simulink model "Scope1"  (R2025b)
settings: Solver=VariableStepAuto  StartTime=0.0  StopTime=10.0  RelTol=1e-3
libraries: simulink x1
settings Model: Creator=fmarini  LastModifiedBy=Claudia Yasar
settings SolverCC: AlgebraicLoopSolver=TrustRegion
settings DebuggingCC: UnconnectedInputMsg=warning  UnconnectedOutputMsg=warning  UnconnectedLineMsg=warning
settings ModelReferenceCC: EnableRefExpFcnMdlSchedulingChecks=on
settings RTWCC: GPUComputeCapability=3.5

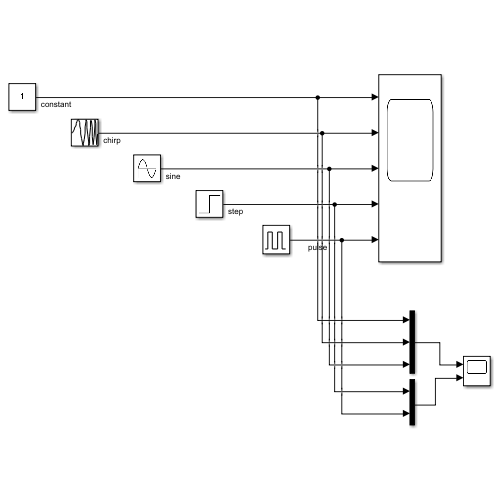
[thumbnail: Simulink's stored preview of the top-level diagram]
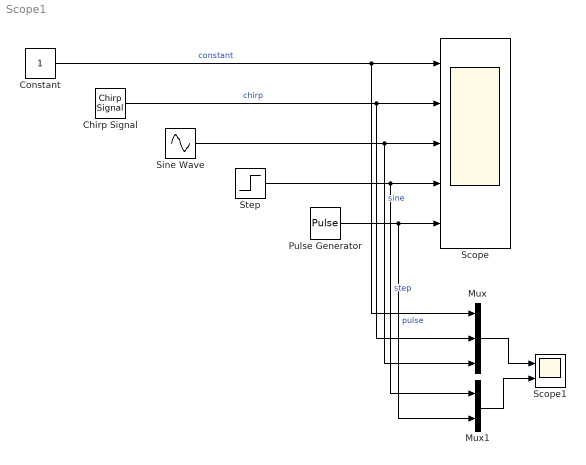
== system Scope1 ==
  Chirp Signal : simulink/Sources/Chirp Signal  f1=0.1  T=100  f2=1
  Constant : Constant
  Mux : Mux  Inputs=3
  Mux1 : Mux  Inputs=2
  Pulse Generator : DiscretePulseGenerator  PulseType=Time based  PulseWidth=5
  Scope : Scope  NumInputPorts=5
      settings: ActiveDisplayYMinimum=-1.24991  ActiveDisplayYMaximum=1.24999
  Scope1 : Scope  NumInputPorts=2
      settings: ActiveDisplayYMinimum=-1.24991  ActiveDisplayYMaximum=1.24999
  Sine Wave : Sin  SampleTime=0
  Step : Step  SampleTime=0.1
  wires:
  Sine Wave/1 -> Mux/3, Scope/3  "sine"
  Step/1 -> Mux1/1, Scope/4  "step"
  Pulse Generator/1 -> Mux1/2, Scope/5  "pulse"
  Chirp Signal/1 -> Mux/2, Scope/2  "chirp"
  Constant/1 -> Mux/1, Scope/1  "constant"
  Mux/1 -> Scope1/1
  Mux1/1 -> Scope1/2
